simulink model "TailsitterSimModel_INDI_simple"  (R2018b)
settings: Solver=ode45  StartTime=0  StopTime=1200  FixedStep=0.001  RelTol=1e-4  EnableMultiTasking=on
undefined symbols (not defined in the file): jystck, sigbuilder_block
libraries: unit_conversions_lib x3, tailsitter_lib x2, aerolibfltsims x2, axes_transformation_lib x1, fmCopterAttiRedIndi_lib x1, aerolibanimutils x1, atmosphere_lib x1, joystick_lib x1
settings Model: Creator=Yannic  LastModifiedBy=yannic
settings SolverCC: ZeroCrossControl=DisableAll  AlgebraicLoopSolver=LineSearch
settings DataIOCC: LimitDataPoints=on  SaveFormat=StructureWithTime
settings OptimizationCC: BlockReduction=off  DefaultParameterBehavior=Inlined  OptimizeBlockIOStorage=off  BufferReuse=off  GlobalBufferReuse=off  ExpressionFolding=off  LocalBlockOutputs=off  LifeSpan=inf  OptimizeDataStoreBuffers=off  BusAssignmentInplaceUpdate=off
settings DebuggingCC: AlgebraicLoopMsg=none  UnconnectedInputMsg=none  UnconnectedOutputMsg=none  UnconnectedLineMsg=none  AllowSymbolicDim=off  SFUnexpectedBacktrackingDiag=warning  SFNoUnconditionalDefaultTransitionDiag=warning  SFExecutionAtInitializationDiag=none
settings ModelReferenceCC: PropagateSignalLabelsOutOfModel=off
settings SFSimCC: SimUseLocalCustomCode=off
settings RTWCC: RTWUseLocalCustomCode=off
settings CodeAppCC: StateflowObjectComments=on
settings GRTTargetCC: TargetLangStandard=C89/C90 (ANSI)
settings ConfigComp: CovMetricSettings=dw  CovHtmlReporting=on  CovSaveCumulativeToWorkspaceVar=on  CovSaveSingleToWorkspaceVar=on  CovExternalEMLEnable=off

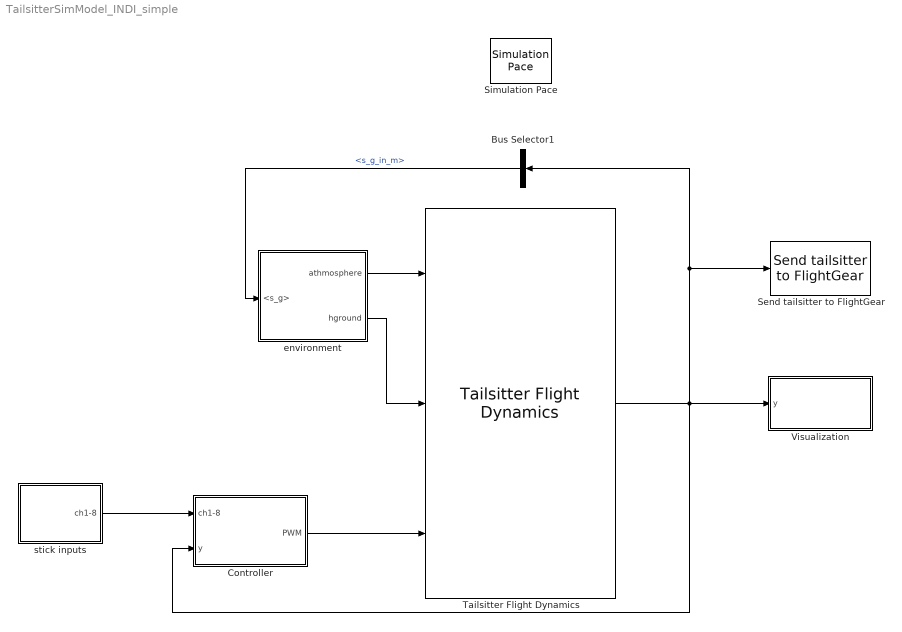
== system TailsitterSimModel_INDI_simple ==
  Bus Selector1 : BusSelector  OutputSignals=rigid_body.s_g_in_m
  Controller : Subsystem
  Send tailsitter to FlightGear : tailsitter_lib/Send tailsitter to FlightGear  posRef=tailsitter.posRef  IP='127.0.0.1'  Port=5502
      settings: SourceProductName=LADAC
  Simulation Pace : aerolibanimutils/Simulation Pace  SimulationPace=pace  SleepMode=MATLAB Thread  OutputPaceError=off  SampleTime=1/30
  Tailsitter Flight Dynamics : tailsitter_lib/Tailsitter Flight Dynamics  tailsitter=tailsitter
      settings: SourceProductName=LADAC
  Visualization : Subsystem
  environment : Subsystem
  stick inputs : Subsystem
  wires:
  environment/1(athmosphere) -> Tailsitter Flight Dynamics/1
  environment/2(hground) -> Tailsitter Flight Dynamics/2
  Tailsitter Flight Dynamics/1 -> Send tailsitter to FlightGear/1, Bus Selector1/1, Visualization/1(y), Controller/2(y)
  Bus Selector1/1 -> environment/1(<s_g>)  "<s_g_in_m>"
  stick inputs/1(ch1-8) -> Controller/1(ch1-8)
  Controller/1(PWM) -> Tailsitter Flight Dynamics/3

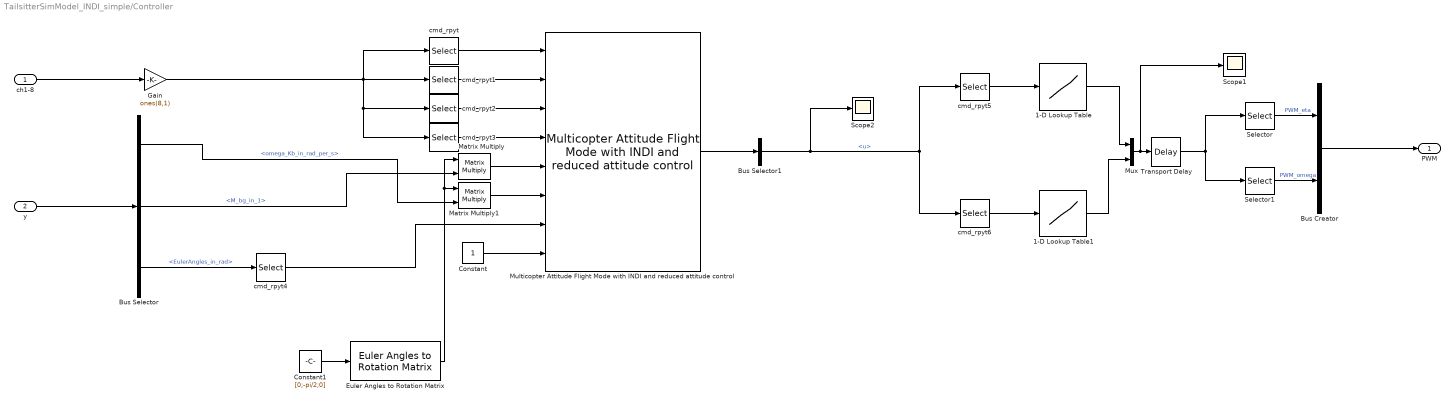
== system TailsitterSimModel_INDI_simple/Controller ==
  ch1-8 : Inport  OutDataTypeStr=double
  y : Inport  Port=2
  1-D Lookup Table : Lookup_n-D  NumberOfTableDimensions=1  BreakpointsForDimension1=[0,1]  Table=[1100,1900]  InternalRulePriority=Speed  RndMeth=Simplest  InputSameDT=on
  1-D Lookup Table1 : Lookup_n-D  NumberOfTableDimensions=1  BreakpointsForDimension1=[0,1]  Table=[1000,2000]  InternalRulePriority=Speed  RndMeth=Simplest  InputSameDT=on
  Bus Creator : BusCreator  Inputs=2
  Bus Selector : BusSelector  OutputSignals=rigid_body.omega_Kb_in_rad_per_s,rigid_body.M_bg_in_1,rigid_body.EulerAngles_in_rad
  Bus Selector1 : BusSelector  OutputSignals=u
  Constant : Constant  OutDataTypeStr=Inherit: Inherit via back propagation
  Constant1 : Constant  Value=[0;-pi/2;0]  OutDataTypeStr=Inherit: Inherit via back propagation
  Euler Angles to Rotation Matrix : axes_transformation_lib/Euler Angles to Rotation Matrix  SystemSampleTime=-1
      settings: SourceProductName=LADAC
  Gain : Gain  Gain=ones(8,1)
  Matrix Multiply : Product  Multiplication=Matrix(*)
  Matrix Multiply1 : Product  Multiplication=Matrix(*)
  Multicopter Attitude Flight Mode with INDI and reduced attitude control : fmCopterAttiRedIndi_lib/Multicopter Attitude Flight Mode with INDI and reduced attitude control  fm=fm_atti
      settings: SourceProductName=LADAC
  Mux : Mux  Inputs=2
  Scope1 : Scope
  Scope2 : Scope
  Selector : Selector  InputPortWidth=4  IndexOptions=Index vector (dialog)  Indices=[1:2]  OutputSizes=1
  Selector1 : Selector  InputPortWidth=4  IndexOptions=Index vector (dialog)  Indices=[3:4]  OutputSizes=1
  Transport Delay : TransportDelay  DelayTime=0.01*0
  cmd_rpyt : Selector  InputPortWidth=8  IndexOptions=Index vector (dialog)  Indices=1  OutputSizes=1
  cmd_rpyt1 : Selector  InputPortWidth=8  IndexOptions=Index vector (dialog)  Indices=2  OutputSizes=1
  cmd_rpyt2 : Selector  InputPortWidth=8  IndexOptions=Index vector (dialog)  Indices=3  OutputSizes=1
  cmd_rpyt3 : Selector  InputPortWidth=8  IndexOptions=Index vector (dialog)  Indices=4  OutputSizes=1
  cmd_rpyt4 : Selector  InputPortWidth=3  IndexOptions=Index vector (dialog)  Indices=3  OutputSizes=1
  cmd_rpyt5 : Selector  InputPortWidth=4  IndexOptions=Index vector (dialog)  Indices=[1,2]  OutputSizes=1
  cmd_rpyt6 : Selector  InputPortWidth=4  IndexOptions=Index vector (dialog)  Indices=[3,4]  OutputSizes=1
  PWM : Outport
  wires:
  y/1 -> Bus Selector/1
  Selector/1 -> Bus Creator/1  "PWM_eta"
  Selector1/1 -> Bus Creator/2  "PWM_omega"
  Bus Creator/1 -> PWM/1
  Bus Selector/1 -> Matrix Multiply1/2  "<omega_Kb_in_rad_per_s>"
  Bus Selector/2 -> Matrix Multiply/2  "<M_bg_in_1>"
  ch1-8/1 -> Gain/1
  Gain/1 -> cmd_rpyt3/1, cmd_rpyt2/1, cmd_rpyt1/1, cmd_rpyt/1
  Bus Selector1/1 -> cmd_rpyt6/1, cmd_rpyt5/1, Scope2/1  "<u>"
  cmd_rpyt/1 -> Multicopter Attitude Flight Mode with INDI and reduced attitude control/1
  Transport Delay/1 -> Selector1/1, Selector/1
  cmd_rpyt1/1 -> Multicopter Attitude Flight Mode with INDI and reduced attitude control/2
  cmd_rpyt2/1 -> Multicopter Attitude Flight Mode with INDI and reduced attitude control/3
  cmd_rpyt3/1 -> Multicopter Attitude Flight Mode with INDI and reduced attitude control/4
  Bus Selector/3 -> cmd_rpyt4/1  "<EulerAngles_in_rad>"
  Constant/1 -> Multicopter Attitude Flight Mode with INDI and reduced attitude control/8
  Multicopter Attitude Flight Mode with INDI and reduced attitude control/1 -> Bus Selector1/1
  1-D Lookup Table/1 -> Mux/1
  cmd_rpyt5/1 -> 1-D Lookup Table/1
  cmd_rpyt6/1 -> 1-D Lookup Table1/1
  Mux/1 -> Scope1/1, Transport Delay/1
  1-D Lookup Table1/1 -> Mux/2
  cmd_rpyt4/1 -> Multicopter Attitude Flight Mode with INDI and reduced attitude control/7
  Constant1/1 -> Euler Angles to Rotation Matrix/1
  Matrix Multiply/1 -> Multicopter Attitude Flight Mode with INDI and reduced attitude control/5
  Euler Angles to Rotation Matrix/1 -> Matrix Multiply1/1, Matrix Multiply/1
  Matrix Multiply1/1 -> Multicopter Attitude Flight Mode with INDI and reduced attitude control/6

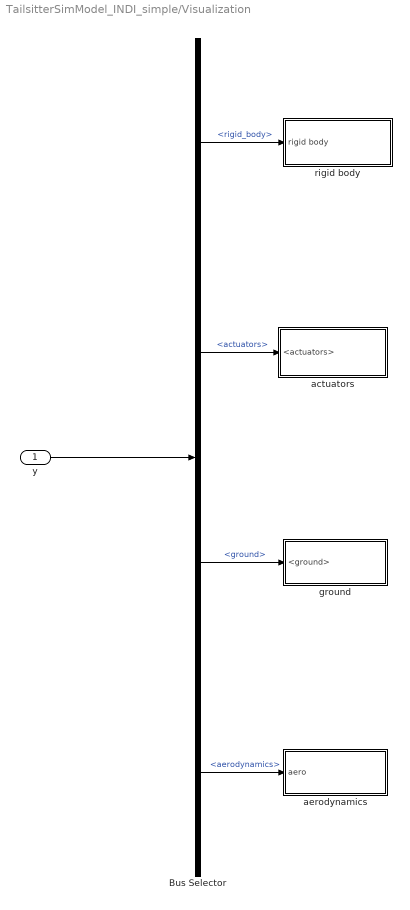
== system TailsitterSimModel_INDI_simple/Visualization ==
  y : Inport
  Bus Selector : BusSelector  OutputSignals=rigid_body,actuators,ground,aerodynamics
  actuators : Subsystem
  aerodynamics : Subsystem
  ground : Subsystem
  rigid body : Subsystem
  wires:
  Bus Selector/1 -> rigid body/1(rigid body)  "<rigid_body>"
  y/1 -> Bus Selector/1
  Bus Selector/4 -> aerodynamics/1(aero)  "<aerodynamics>"
  Bus Selector/3 -> ground/1(<ground>)  "<ground>"
  Bus Selector/2 -> actuators/1(<actuators>)  "<actuators>"

== system TailsitterSimModel_INDI_simple/environment ==
  <s_g> : Inport
  Atmosphere1 : Subsystem
  From FlightGear : Subsystem
  athmosphere : Outport
  hground : Outport  Port=2
  wires:
  From FlightGear/1(hground) -> hground/1
  Atmosphere1/1(atmosphere) -> athmosphere/1
  <s_g>/1 -> Atmosphere1/1(s_g)

== system TailsitterSimModel_INDI_simple/stick inputs ==
  Calibrated Joystick : joystick_lib/Calibrated Joystick  jystck=jystck
      settings: SourceProductName=LADAC
  Constant2 : Constant  Value=jystck.enable
  Scope : Scope
  Signal builder : Subsystem
  Switch : Switch  Criteria=u2 > Threshold
  ch1-8 : Outport
  wires:
  Constant2/1 -> Calibrated Joystick/Enable, Switch/2
  Signal builder/1(r) -> Switch/3
  Calibrated Joystick/1 -> Switch/1
  Switch/1 -> ch1-8/1, Scope/1

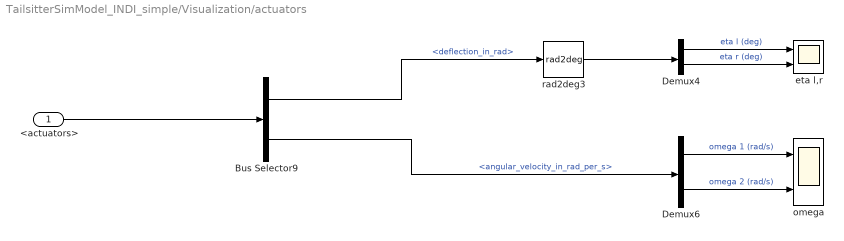
== system TailsitterSimModel_INDI_simple/Visualization/actuators ==
  <actuators> : Inport
  Bus Selector9 : BusSelector  OutputSignals=eta_i.deflection_in_rad,angular_velocity_in_rad_per_s
  Demux4 : Demux  Outputs=2
  Demux6 : Demux  Outputs=2
  eta l,r : Scope  NumInputPorts=2
  omega : Scope  NumInputPorts=2
  rad2deg3 : unit_conversions_lib/rad2deg
      settings: SourceProductName=LADAC
  wires:
  Bus Selector9/1 -> rad2deg3/1  "<deflection_in_rad>"
  Demux4/1 -> eta l,r/1  "eta l (deg)"
  <actuators>/1 -> Bus Selector9/1
  Demux6/2 -> omega/2  "omega 2 (rad/s)"
  Demux4/2 -> eta l,r/2  "eta r (deg)"
  rad2deg3/1 -> Demux4/1
  Demux6/1 -> omega/1  "omega 1 (rad/s)"
  Bus Selector9/2 -> Demux6/1  "<angular_velocity_in_rad_per_s>"

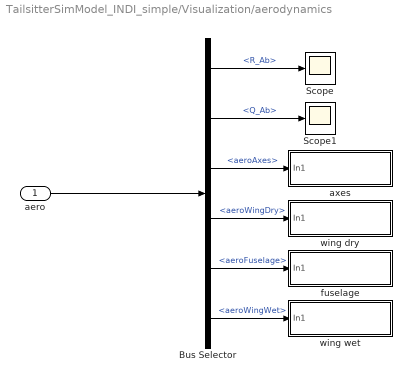
== system TailsitterSimModel_INDI_simple/Visualization/aerodynamics ==
  aero : Inport
  Bus Selector : BusSelector  OutputSignals=cg aerodynamics.R_Ab,cg aerodynamics.Q_Ab,cg aerodynamics.aeroAxes,local aerodynamic.aeroWingDry,local aerodynamic.aeroFuselage,local aerodynamic.aeroWingWet
  Scope : Scope
  Scope1 : Scope
  axes : Subsystem
  fuselage : Subsystem
  wing dry : Subsystem
  wing wet : Subsystem
  wires:
  aero/1 -> Bus Selector/1
  Bus Selector/1 -> Scope/1  "<R_Ab>"
  Bus Selector/2 -> Scope1/1  "<Q_Ab>"
  Bus Selector/3 -> axes/1(In1)  "<aeroAxes>"
  Bus Selector/4 -> wing dry/1(In1)  "<aeroWingDry>"
  Bus Selector/5 -> fuselage/1(In1)  "<aeroFuselage>"
  Bus Selector/6 -> wing wet/1(In1)  "<aeroWingWet>"

== system TailsitterSimModel_INDI_simple/Visualization/ground ==
  <ground> : Inport
  Bus Selector1 : BusSelector  Commented=on  OutputSignals=R_Gb,Q_Gb,alt_hitpoints,e_z
  Scope{1..4} (4 alike) : Scope  Commented=on
  wires:
  <ground>/1 -> Bus Selector1/1
  Bus Selector1/2 -> Scope2/1  "<Q_Gb>"
  Bus Selector1/3 -> Scope3/1  "<alt_hitpoints>"
  Bus Selector1/1 -> Scope1/1  "<R_Gb>"
  Bus Selector1/4 -> Scope4/1  "<e_z>"

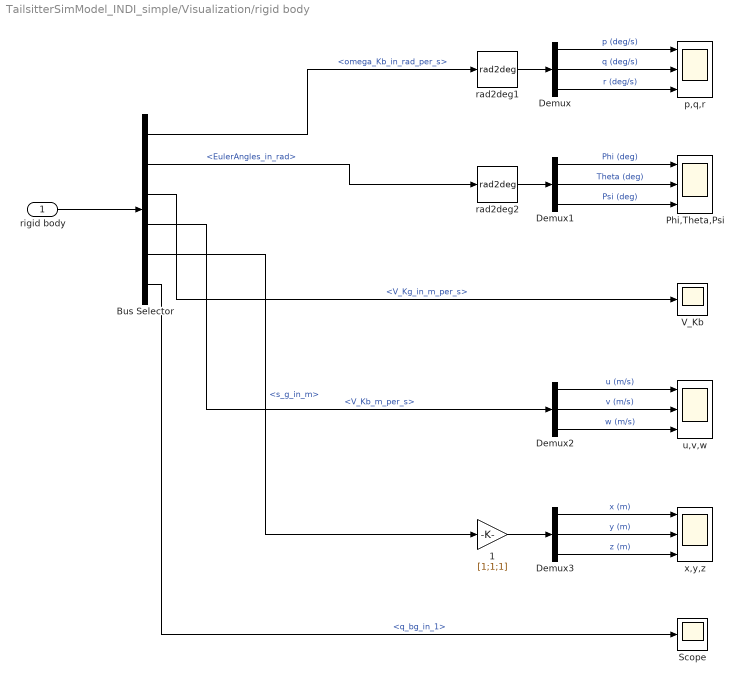
== system TailsitterSimModel_INDI_simple/Visualization/rigid body ==
  rigid body : Inport
  1 : Gain  Gain=[1;1;1]
  Bus Selector : BusSelector  OutputSignals=omega_Kb_in_rad_per_s,EulerAngles_in_rad,V_Kg_in_m_per_s,V_Kb_m_per_s,s_g_in_m,q_bg_in_1
  Demux{,1..3} (4 alike) : Demux  Outputs=3
  Phi,Theta,Psi : Scope  NumInputPorts=3
  Scope : Scope
  V_Kb : Scope
  p,q,r : Scope  NumInputPorts=3
  rad2deg1 : unit_conversions_lib/rad2deg
      settings: SourceProductName=LADAC
  rad2deg2 : unit_conversions_lib/rad2deg
      settings: SourceProductName=LADAC
  u,v,w : Scope  NumInputPorts=3
  x,y,z : Scope  NumInputPorts=3
  wires:
  rad2deg2/1 -> Demux1/1
  Demux1/3 -> Phi,Theta,Psi/3  "Psi (deg)"
  Demux/3 -> p,q,r/3  "r (deg/s)"
  Demux2/2 -> u,v,w/2  "v (m/s)"
  Demux3/1 -> x,y,z/1  "x (m)"
  Demux2/3 -> u,v,w/3  "w (m/s)"
  rad2deg1/1 -> Demux/1
  Demux/2 -> p,q,r/2  "q (deg/s)"
  Demux2/1 -> u,v,w/1  "u (m/s)"
  Demux/1 -> p,q,r/1  "p (deg/s)"
  1/1 -> Demux3/1
  Bus Selector/3 -> V_Kb/1  "<V_Kg_in_m_per_s>"
  Demux1/2 -> Phi,Theta,Psi/2  "Theta (deg)"
  Demux3/2 -> x,y,z/2  "y (m)"
  Demux3/3 -> x,y,z/3  "z (m)"
  Demux1/1 -> Phi,Theta,Psi/1  "Phi (deg)"
  rigid body/1 -> Bus Selector/1
  Bus Selector/1 -> rad2deg1/1  "<omega_Kb_in_rad_per_s>"
  Bus Selector/2 -> rad2deg2/1  "<EulerAngles_in_rad>"
  Bus Selector/4 -> Demux2/1  "<V_Kb_m_per_s>"
  Bus Selector/5 -> 1/1  "<s_g_in_m>"
  Bus Selector/6 -> Scope/1  "<q_bg_in_1>"

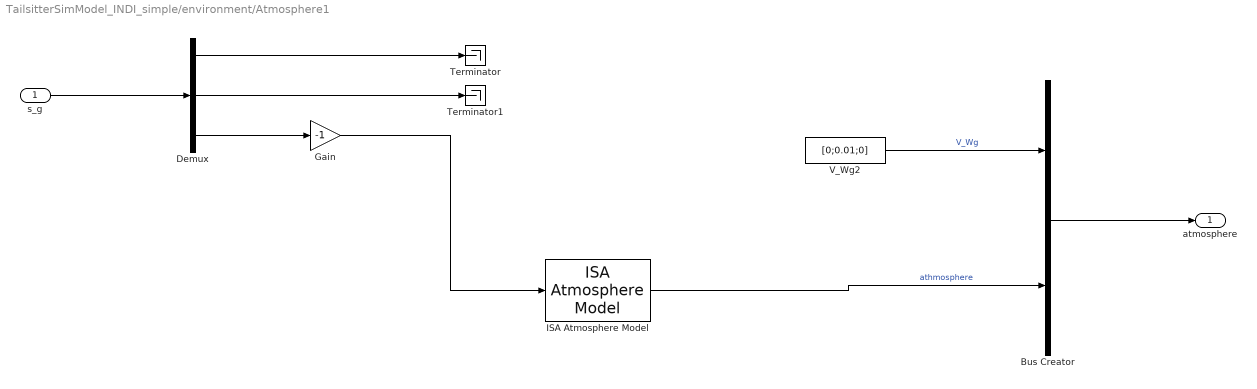
== system TailsitterSimModel_INDI_simple/environment/Atmosphere1 ==
  s_g : Inport
  Bus Creator : BusCreator  Inputs=2
  Demux : Demux  Outputs=3
  Gain : Gain  Gain=-1
  ISA Atmosphere Model : atmosphere_lib/ISA Atmosphere Model  SystemSampleTime=-1
      settings: SourceProductName=LADAC
  Terminator : Terminator
  Terminator1 : Terminator
  V_Wg2 : Constant  Value=[0;0.01;0]
  atmosphere : Outport
  wires:
  ISA Atmosphere Model/1 -> Bus Creator/2  "athmosphere"
  Demux/1 -> Terminator/1
  Demux/2 -> Terminator1/1
  s_g/1 -> Demux/1
  Demux/3 -> Gain/1
  Gain/1 -> ISA Atmosphere Model/1
  Bus Creator/1 -> atmosphere/1
  V_Wg2/1 -> Bus Creator/1  "V_Wg"

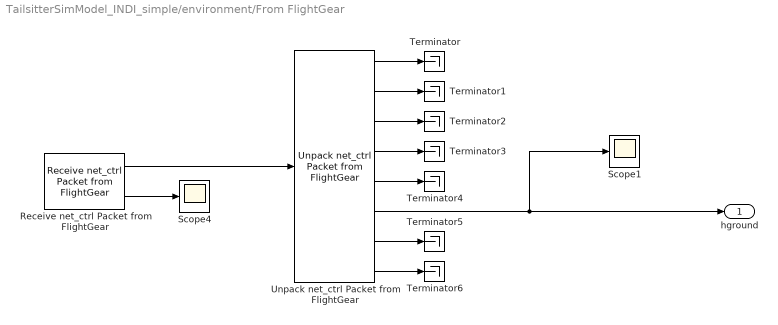
== system TailsitterSimModel_INDI_simple/environment/From FlightGear ==
  Receive net_ctrl Packet from FlightGear : aerolibfltsims/Receive net_ctrl Packet from FlightGear  FlightGearVersion=v3.4  ReceiveAddress=127.0.0.1  ReceivePort=5503  ReceiveWidth=744  varLen=off  SampleTime=1/30  packetFlag=on
      settings: AttributesFormatString=Version Selected:\n%<FlightGearVersion>  SourceProductName=Aerospace Blockset  SourceProductBaseCode=AE
  Scope1 : Scope
  Scope4 : Scope
  Terminator{,1..6} (7 alike) : Terminator
  Unpack net_ctrl Packet from FlightGear : aerolibfltsims/Unpack net_ctrl Packet from FlightGear  FlightGearVersion=v3.4  ShowControlSurfacePositionOutputs=off  ShowEngineFuelOutputs=off  ShowLandingGearOutputs=off  ShowAvionicOutputs=off  ShowEnvironmentOutputs=on  SampleTime=1/30  packetVersion=27
      settings: AttributesFormatString=Version Selected: %<FlightGearVersion>  SourceProductName=Aerospace Blockset  SourceProductBaseCode=AE
  hground : Outport
  wires:
  Receive net_ctrl Packet from FlightGear/2 -> Scope4/1
  Unpack net_ctrl Packet from FlightGear/5 -> Terminator4/1
  Unpack net_ctrl Packet from FlightGear/4 -> Terminator3/1
  Unpack net_ctrl Packet from FlightGear/2 -> Terminator1/1
  Receive net_ctrl Packet from FlightGear/1 -> Unpack net_ctrl Packet from FlightGear/1
  Unpack net_ctrl Packet from FlightGear/1 -> Terminator/1
  Unpack net_ctrl Packet from FlightGear/8 -> Terminator6/1
  Unpack net_ctrl Packet from FlightGear/6 -> Scope1/1, hground/1
  Unpack net_ctrl Packet from FlightGear/3 -> Terminator2/1
  Unpack net_ctrl Packet from FlightGear/7 -> Terminator5/1

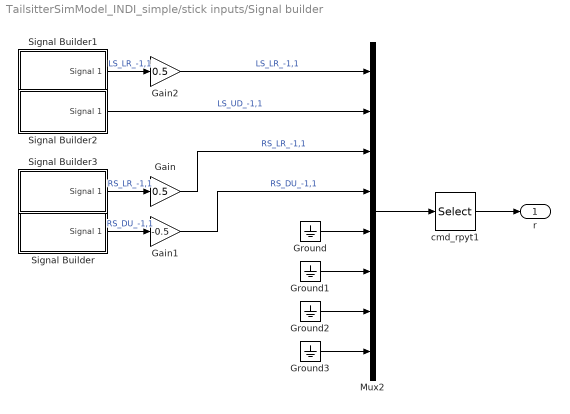
== system TailsitterSimModel_INDI_simple/stick inputs/Signal builder ==
  Gain : Gain  Gain=0.5
  Gain1 : Gain  Gain=-0.5
  Gain2 : Gain  Gain=0.5
  Ground{,1..3} (4 alike) : Ground
  Mux2 : Mux  Inputs=8
  Signal Builder : Subsystem  Tag=STV Subsys  LoadFcn=sigbuilder_block('load');  StartFcn=sigbuilder_block('start');  StopFcn=sigbuilder_block('stop');  ClipboardFcn=sigbuilder_block('clipboard');  mask(Sigbuilder block){tuvar=[0:10]}
      mask help: Simulink:masks:SigbuilderBlock_MD
      mask init:
      | if ~strcmp(get_param(bdroot(gcbh),'SimulationStatus'),'stopped') tuvar = sigbuilder_block('maskInit'); end
      settings: CopyFcn=sigbuilder_block('copy');  DeleteFcn=sigbuilder_block('delete');  ModelCloseFcn=sigbuilder_block('modelClose');  PreSaveFcn=sigbuilder_block('preSave');  PauseFcn=sigbuilder_block('pause');  ContinueFcn=sigbuilder_block('continue');  NameChangeFcn=sigbuilder_block('namechange');  OpenFcn=sigbuilder_block('open',[426 42.75 821.25 509.25 ]);  CloseFcn=sigbuilder_block('close');
      mask Display: plot(0, 0, 100, 100,[2, 2, 32, 32, 2], [68, 8, 8, 68, 68],[32, 2], [38, 38], [32, 19, 2],[53, 60, 44], [32, 17, 17, 2],[16, 16, 31, 31]);txt = getActiveGroup(gcbh);text(2, 100, txt,'verticalAlignment', 'top');
  Signal Builder1 : Subsystem  Tag=STV Subsys  LoadFcn=sigbuilder_block('load');  StartFcn=sigbuilder_block('start');  StopFcn=sigbuilder_block('stop');  ClipboardFcn=sigbuilder_block('clipboard');  mask(Sigbuilder block){tuvar=[0:10]}
      mask help: Simulink:masks:SigbuilderBlock_MD
      mask init:
      | if ~strcmp(get_param(bdroot(gcbh),'SimulationStatus'),'stopped') tuvar = sigbuilder_block('maskInit'); end
      settings: CopyFcn=sigbuilder_block('copy');  DeleteFcn=sigbuilder_block('delete');  ModelCloseFcn=sigbuilder_block('modelClose');  PreSaveFcn=sigbuilder_block('preSave');  PauseFcn=sigbuilder_block('pause');  ContinueFcn=sigbuilder_block('continue');  NameChangeFcn=sigbuilder_block('namechange');  OpenFcn=sigbuilder_block('open',[429.75 123 565.5 444.75 ]);  CloseFcn=sigbuilder_block('close');
      mask Display: plot(0, 0, 100, 100,[2, 2, 32, 32, 2], [68, 8, 8, 68, 68],[32, 2], [38, 38], [32, 19, 2],[53, 60, 44], [32, 17, 17, 2],[16, 16, 31, 31]);txt = getActiveGroup(gcbh);text(2, 100, txt,'verticalAlignment', 'top');
  Signal Builder2 : Subsystem  Tag=STV Subsys  LoadFcn=sigbuilder_block('load');  StartFcn=sigbuilder_block('start');  StopFcn=sigbuilder_block('stop');  ClipboardFcn=sigbuilder_block('clipboard');  mask(Sigbuilder block){tuvar=[0:10]}
      mask help: Simulink:masks:SigbuilderBlock_MD
      mask init:
      | if ~strcmp(get_param(bdroot(gcbh),'SimulationStatus'),'stopped') tuvar = sigbuilder_block('maskInit'); end
      settings: CopyFcn=sigbuilder_block('copy');  DeleteFcn=sigbuilder_block('delete');  ModelCloseFcn=sigbuilder_block('modelClose');  PreSaveFcn=sigbuilder_block('preSave');  PauseFcn=sigbuilder_block('pause');  ContinueFcn=sigbuilder_block('continue');  NameChangeFcn=sigbuilder_block('namechange');  OpenFcn=sigbuilder_block('open',[411 0 603 557.25 ]);  CloseFcn=sigbuilder_block('close');
      mask Display: plot(0, 0, 100, 100,[2, 2, 32, 32, 2], [68, 8, 8, 68, 68],[32, 2], [38, 38], [32, 19, 2],[53, 60, 44], [32, 17, 17, 2],[16, 16, 31, 31]);txt = getActiveGroup(gcbh);text(2, 100, txt,'verticalAlignment', 'top');
  Signal Builder3 : Subsystem  Tag=STV Subsys  LoadFcn=sigbuilder_block('load');  StartFcn=sigbuilder_block('start');  StopFcn=sigbuilder_block('stop');  ClipboardFcn=sigbuilder_block('clipboard');  mask(Sigbuilder block){tuvar=[0:10]}
      mask help: Simulink:masks:SigbuilderBlock_MD
      mask init:
      | if ~strcmp(get_param(bdroot(gcbh),'SimulationStatus'),'stopped') tuvar = sigbuilder_block('maskInit'); end
      settings: CopyFcn=sigbuilder_block('copy');  DeleteFcn=sigbuilder_block('delete');  ModelCloseFcn=sigbuilder_block('modelClose');  PreSaveFcn=sigbuilder_block('preSave');  PauseFcn=sigbuilder_block('pause');  ContinueFcn=sigbuilder_block('continue');  NameChangeFcn=sigbuilder_block('namechange');  OpenFcn=sigbuilder_block('open',[433.5 161.25 558 422.25 ]);  CloseFcn=sigbuilder_block('close');
      mask Display: plot(0, 0, 100, 100,[2, 2, 32, 32, 2], [68, 8, 8, 68, 68],[32, 2], [38, 38], [32, 19, 2],[53, 60, 44], [32, 17, 17, 2],[16, 16, 31, 31]);txt = getActiveGroup(gcbh);text(2, 100, txt,'verticalAlignment', 'top');
  cmd_rpyt1 : Selector  InputPortWidth=8  IndexOptions=Index vector (dialog)  Indices=[3,4,1,2,5,6,7,8]  OutputSizes=1
  r : Outport
  wires:
  Ground3/1 -> Mux2/8
  Gain2/1 -> Mux2/1  "LS_LR_-1,1"
  Ground1/1 -> Mux2/6
  Ground2/1 -> Mux2/7
  Mux2/1 -> cmd_rpyt1/1
  Signal Builder2/1(Signal 1) -> Mux2/2  "LS_UD_-1,1"
  Gain/1 -> Mux2/3  "RS_LR_-1,1"
  Ground/1 -> Mux2/5
  Gain1/1 -> Mux2/4  "RS_DU_-1,1"
  Signal Builder3/1(Signal 1) -> Gain/1  "RS_LR_-1,1"
  Signal Builder/1(Signal 1) -> Gain1/1  "RS_DU_-1,1"
  Signal Builder1/1(Signal 1) -> Gain2/1  "LS_LR_-1,1"
  cmd_rpyt1/1 -> r/1

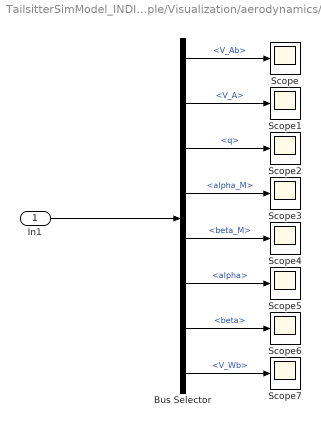
== system TailsitterSimModel_INDI_simple/Visualization/aerodynamics/axes ==
  In1 : Inport
  Bus Selector : BusSelector  OutputSignals=V_Ab,V_A,q,alpha_M,beta_M,alpha,beta,V_Wb
  Scope{,1..7} (8 alike) : Scope
  wires:
  In1/1 -> Bus Selector/1
  Bus Selector/1 -> Scope/1  "<V_Ab>"
  Bus Selector/2 -> Scope1/1  "<V_A>"
  Bus Selector/3 -> Scope2/1  "<q>"
  Bus Selector/4 -> Scope3/1  "<alpha_M>"
  Bus Selector/5 -> Scope4/1  "<beta_M>"
  Bus Selector/6 -> Scope5/1  "<alpha>"
  Bus Selector/7 -> Scope6/1  "<beta>"
  Bus Selector/8 -> Scope7/1  "<V_Wb>"

== system TailsitterSimModel_INDI_simple/Visualization/aerodynamics/fuselage ==
  In1 : Inport
  Bus Selector : BusSelector  OutputSignals=aeroAxes,dynamics
  wing weet : Subsystem
  wing weet1 : Subsystem
  wires:
  In1/1 -> Bus Selector/1
  Bus Selector/1 -> wing weet/1(In1)  "<aeroAxes>"
  Bus Selector/2 -> wing weet1/1(In1)  "<dynamics>"

== system TailsitterSimModel_INDI_simple/Visualization/aerodynamics/wing dry ==
  In1 : Inport
  Bus Selector : BusSelector  OutputSignals=aeroAxes,dynamicsBody
  axes : Subsystem
  dynamics : Subsystem
  wires:
  In1/1 -> Bus Selector/1
  Bus Selector/2 -> dynamics/1(In1)  "<dynamicsBody>"
  Bus Selector/1 -> axes/1(In1)  "<aeroAxes>"

== system TailsitterSimModel_INDI_simple/Visualization/aerodynamics/wing wet ==
  In1 : Inport
  Bus Selector : BusSelector  OutputSignals=dynamicsBody,aeroAxes
  axes : Subsystem
  dynamics : Subsystem
  wires:
  In1/1 -> Bus Selector/1
  Bus Selector/1 -> dynamics/1(In1)  "<dynamicsBody>"
  Bus Selector/2 -> axes/1(In1)  "<aeroAxes>"

== system TailsitterSimModel_INDI_simple/stick inputs/Signal builder/Signal Builder ==
  Demux : Demux  Tag=STV Demux  Outputs=1
  FromWs : FromWorkspace  Tag=STV FromWs  VariableName=tuvar  SampleTime=0
      SigBuilderData=|
      | common.afterFinalStr = 'Extrapolate'
      | common.sampleTime = 0
      | dataSet.timeRange = [0 10]
      | dataSet.name = 'Group 1'
      | sbobj.Groups.Name = 'Group 1'
      | sbobj.Groups.Signals.Name = 'Signal 1'
      | sbobj.Groups.Signals.XData = [0 8 8 9.9 9.9 9.92 9.92 9.96 9.96 10]
      | sbobj.Groups.Signals.YData = [0 0 1 1 1.005 0.803 0.8 0.4 0 0]
  Signal 1 : Outport  Tag=STV Outport
  wires:
  Demux/1 -> Signal 1/1
  FromWs/1 -> Demux/1

== system TailsitterSimModel_INDI_simple/stick inputs/Signal builder/Signal Builder1 ==
  Demux : Demux  Tag=STV Demux  Outputs=1
  FromWs : FromWorkspace  Tag=STV FromWs  VariableName=tuvar  SampleTime=0
      SigBuilderData=|
      | common.afterFinalStr = 'Extrapolate'
      | common.sampleTime = 0
      | dataSet.timeRange = [0 10]
      | dataSet.name = 'Group 1'
      | sbobj.Groups.Name = 'Group 1'
      | sbobj.Groups.Signals.Name = 'Signal 1'
      | sbobj.Groups.Signals.XData = [0 4 4 6 6 10]
      | sbobj.Groups.Signals.YData = [0 0 1 1 0 0]
  Signal 1 : Outport  Tag=STV Outport
  wires:
  Demux/1 -> Signal 1/1
  FromWs/1 -> Demux/1

== system TailsitterSimModel_INDI_simple/stick inputs/Signal builder/Signal Builder2 ==
  Demux : Demux  Tag=STV Demux  Outputs=1
  FromWs : FromWorkspace  Tag=STV FromWs  VariableName=tuvar  SampleTime=0
      SigBuilderData=|
      | common.afterFinalStr = 'Extrapolate'
      | common.sampleTime = 0
      | dataSet.timeRange = [0 10]
      | dataSet.name = 'Group 1'
      | sbobj.Groups.Name = 'Group 1'
      | sbobj.Groups.Signals.Name = 'Signal 1'
      | sbobj.Groups.Signals.XData = [0 2 2 6 8 10]
      | sbobj.Groups.Signals.YData = [0 0 -1 -1 0 0]
  Signal 1 : Outport  Tag=STV Outport
  wires:
  FromWs/1 -> Demux/1
  Demux/1 -> Signal 1/1

== system TailsitterSimModel_INDI_simple/stick inputs/Signal builder/Signal Builder3 ==
  Demux : Demux  Tag=STV Demux  Outputs=1
  FromWs : FromWorkspace  Tag=STV FromWs  VariableName=tuvar  SampleTime=0
      SigBuilderData=|
      | common.afterFinalStr = 'Extrapolate'
      | common.sampleTime = 0
      | dataSet.timeRange = [0 10]
      | dataSet.name = 'Group 1'
      | sbobj.Groups.Name = 'Group 1'
      | sbobj.Groups.Signals.Name = 'Signal 1'
      | sbobj.Groups.Signals.XData = [0 6 6 8 8 10]
      | sbobj.Groups.Signals.YData = [0 0 1 1 0 0]
  Signal 1 : Outport  Tag=STV Outport
  wires:
  Demux/1 -> Signal 1/1
  FromWs/1 -> Demux/1

== system TailsitterSimModel_INDI_simple/Visualization/aerodynamics/fuselage/wing weet ==
  In1 : Inport
  Bus Selector : BusSelector  OutputSignals=V_A_Pfuse,q_Pfuse,alpha_M_Pfuse,beta_M_Pfuse
  Scope{,1..3} (4 alike) : Scope
  wires:
  In1/1 -> Bus Selector/1
  Bus Selector/1 -> Scope/1  "<V_A_Pfuse>"
  Bus Selector/2 -> Scope1/1  "<q_Pfuse>"
  Bus Selector/3 -> Scope2/1  "<alpha_M_Pfuse>"
  Bus Selector/4 -> Scope3/1  "<beta_M_Pfuse>"

== system TailsitterSimModel_INDI_simple/Visualization/aerodynamics/fuselage/wing weet1 ==
  In1 : Inport
  wires:
  In1/1 -> ?

== system TailsitterSimModel_INDI_simple/Visualization/aerodynamics/wing dry/axes ==
  In1 : Inport
  Bus Selector : BusSelector  OutputSignals=V_A_P,q_P,alpha_M_P,beta_M_P
  Scope{,1..3} (4 alike) : Scope
  wires:
  In1/1 -> Bus Selector/1
  Bus Selector/1 -> Scope/1  "<V_A_P>"
  Bus Selector/2 -> Scope1/1  "<q_P>"
  Bus Selector/3 -> Scope2/1  "<alpha_M_P>"
  Bus Selector/4 -> Scope3/1  "<beta_M_P>"

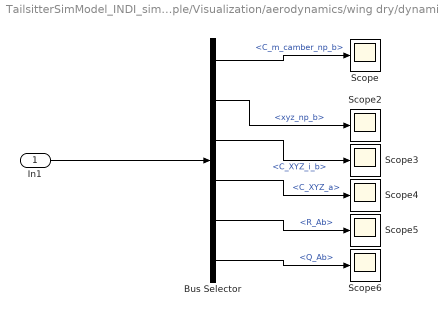
== system TailsitterSimModel_INDI_simple/Visualization/aerodynamics/wing dry/dynamics ==
  In1 : Inport
  Bus Selector : BusSelector  OutputSignals=C_m_camber_np_b,xyz_np_b,C_XYZ_i_b,C_XYZ_a,R_Ab,Q_Ab
  Scope{,2..6} (6 alike) : Scope
  wires:
  In1/1 -> Bus Selector/1
  Bus Selector/1 -> Scope/1  "<C_m_camber_np_b>"
  Bus Selector/2 -> Scope2/1  "<xyz_np_b>"
  Bus Selector/3 -> Scope3/1  "<C_XYZ_i_b>"
  Bus Selector/4 -> Scope4/1  "<C_XYZ_a>"
  Bus Selector/5 -> Scope5/1  "<R_Ab>"
  Bus Selector/6 -> Scope6/1  "<Q_Ab>"

== system TailsitterSimModel_INDI_simple/Visualization/aerodynamics/wing wet/axes ==
  In1 : Inport
  Bus Selector : BusSelector  OutputSignals=V_A_P,q_P,alpha_M_P,beta_M_P
  Scope{,1..3} (4 alike) : Scope
  wires:
  In1/1 -> Bus Selector/1
  Bus Selector/1 -> Scope/1  "<V_A_P>"
  Bus Selector/2 -> Scope1/1  "<q_P>"
  Bus Selector/3 -> Scope2/1  "<alpha_M_P>"
  Bus Selector/4 -> Scope3/1  "<beta_M_P>"

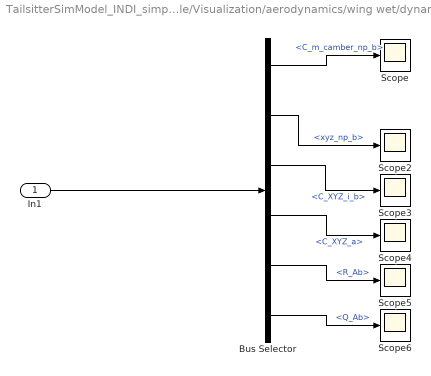
== system TailsitterSimModel_INDI_simple/Visualization/aerodynamics/wing wet/dynamics ==
  In1 : Inport
  Bus Selector : BusSelector  OutputSignals=C_m_camber_np_b,xyz_np_b,C_XYZ_i_b,C_XYZ_a,R_Ab,Q_Ab
  Scope{,2..6} (6 alike) : Scope
  wires:
  In1/1 -> Bus Selector/1
  Bus Selector/1 -> Scope/1  "<C_m_camber_np_b>"
  Bus Selector/2 -> Scope2/1  "<xyz_np_b>"
  Bus Selector/3 -> Scope3/1  "<C_XYZ_i_b>"
  Bus Selector/4 -> Scope4/1  "<C_XYZ_a>"
  Bus Selector/5 -> Scope5/1  "<R_Ab>"
  Bus Selector/6 -> Scope6/1  "<Q_Ab>"
